simulink model "ControllerSimulation"  (R2024a)
settings: Solver=ode45  StartTime=0.0  StopTime=400  RelTol=1e-4
values from neighbouring files (symbols this model uses):
  CpData = [-0.257802999755 -0.378175309838 -0.529522344065 -0.715215887549 -0.938397956285 -1.2018891109 -1.50731652217 -1.85573677772 -2.24586115735 -2.67483575128 -3.1476672426 -3.67843934333 ... (915 elements, 15x61)]    [WindCpData.mat]
undefined symbols (not defined in the file or in its folder): GBEff, GBRatio, GenEff, J_r, K_theta, PRated, R, rho, T_theta, tau, tau_T, WindRated, wRatedLSS
libraries: simulink x2
settings Model: Creator=The MathWorks, Inc.  LastModifiedBy=alber
settings OptimizationCC: ReuseModelBlockBuffer=off
settings DebuggingCC: SubsystemReferenceDiagnosticForUnitTest=warning
settings RTWCC: GPUComputeCapability=3.5

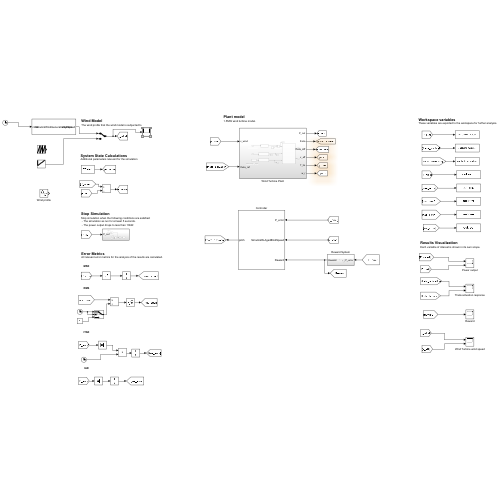
[thumbnail: Simulink's stored preview of the top-level diagram]
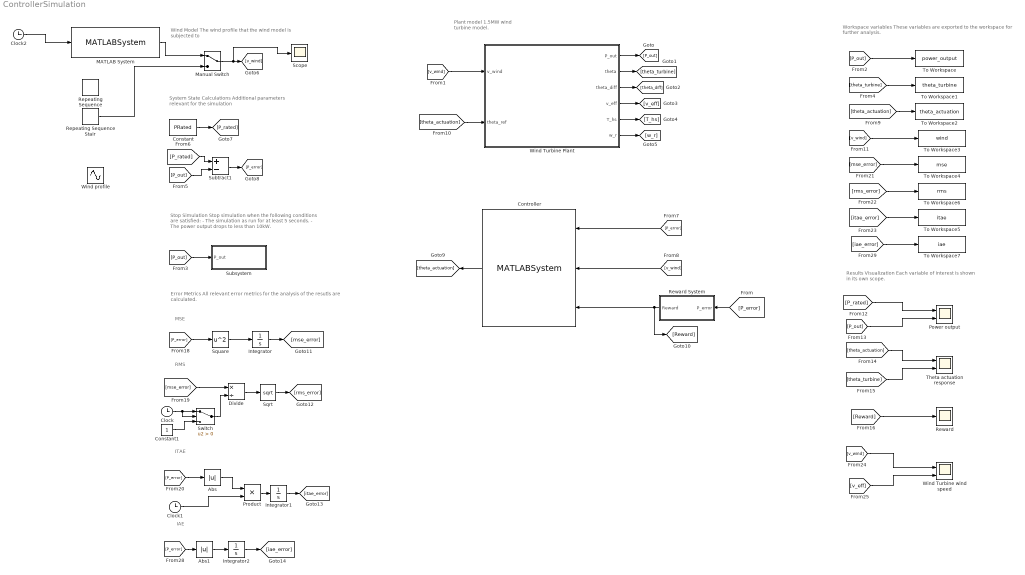
== system ControllerSimulation ==
  note: IAE
  note: MSE
  note: Error Metrics
      | All relevant error metrics for the analysis of the resutls are calculated.
  note: Results Visualization
      | Each variable of interest is shown in its own scope.
  note: System State Calculations
      | Additional parameters relevant for the simulation
  note: Wind Model
      | The wind profile that the wind model is subjected to
  note: Workspace variables
      | These variables are exported to the workspace for further analysis.
  note: Stop Simulation
      | Stop simulation when the following conditions are satisfied:
      | - The simulation as run for at least 5 seconds.
      | - The power output drops to less than 10kW.
  note: Plant model
      | 1.5MW wind turbine model.
  note: RMS
  note: ITAE
  Abs : Abs  SaturateOnIntegerOverflow=off
  Abs1 : Abs  SaturateOnIntegerOverflow=off
  Clock : Clock
  Clock1 : Clock
  Clock2 : Clock
  Constant : Constant  Value=PRated
  Constant1 : Constant
  Controller : MATLABSystem  System=SimulinkRLAgent  SimulateUsing=Interpreted execution
      mask Type: SimulinkRLAgent
      mask Display:
      | disp('SimulinkRLAgent');
      | port_label('input',1,'P_error');
      | port_label('input',2,'WindSpeed');
      | port_label('input',3,'Reward');
      | port_label('output',1,'pitch');
  Divide : Product  Inputs=*/
  Integrator : Integrator
  Integrator1 : Integrator
  Integrator2 : Integrator
  MATLAB System : MATLABSystem  System=SimulinkWindGeneratorSystem  Scale=11.7  Shape=120  Tau=1  MaxRate=0.9  Ts=1  RandomTime=5  SimulateUsing=Interpreted execution
      mask Type: SimulinkWindGeneratorSystem
      mask Display:
      | disp('SimulinkWindGeneratorSystem');
      | port_label('input',1,'clock');
      | port_label('output',1,'windSpeed');
  Manual Switch : ManualSwitch
  Power output : Scope  NumInputPorts=2
  Product : Product
  Repeating Sequence : simulink/Sources/Repeating Sequence  rep_seq_t=[0 401]  rep_seq_y=[11.3 11.9]
  Repeating Sequence Stair : simulink/Sources/Repeating Sequence Stair  OutValues=11.3:0.05:11.9  tsamp=15  OutMin=[11.3]  OutMax=[11.9]  OutDataTypeStr=double  OutputDataTypeScalingMode=double  OutDataType=fixdt(0,8)  ConRadixGroup=Best Precision: Vector-wise  OutScaling=2^-12
  Reward : Scope
  Reward System : Subsystem
  Scope : Scope
  Sqrt : Sqrt
  Square : Math  Operator=square
  Subsystem : Subsystem
  Subtract1 : Sum  Inputs=+-
  Switch : Switch  Criteria=u2 > Threshold  SaturateOnIntegerOverflow=off  InputSameDT=off
  Theta actuation response : Scope  NumInputPorts=2
  To Workspace : ToWorkspace  VariableName=power_output  SaveFormat=Timeseries  SampleTime=-1
  To Workspace1 : ToWorkspace  VariableName=theta_turbine  SaveFormat=Timeseries  SampleTime=-1
  To Workspace2 : ToWorkspace  VariableName=theta_actuation  SaveFormat=Timeseries  SampleTime=-1
  To Workspace3 : ToWorkspace  VariableName=wind  SaveFormat=Timeseries  SampleTime=-1
  To Workspace4 : ToWorkspace  VariableName=mse  SaveFormat=Timeseries  SampleTime=-1
  To Workspace5 : ToWorkspace  VariableName=itae  SaveFormat=Timeseries  SampleTime=-1
  To Workspace6 : ToWorkspace  VariableName=rms  SaveFormat=Timeseries  SampleTime=-1
  To Workspace7 : ToWorkspace  VariableName=iae  SaveFormat=Timeseries  SampleTime=-1
  Wind Turbine Plant : Subsystem
  Wind Turbine wind speed : Scope  NumInputPorts=2
  Wind profile : Sin  Amplitude=.2  Bias=WindRated+0.4  Frequency=0.05  SampleTime=0
  wires:
  Wind Turbine Plant/1(P_out) -> [P_out]
  Wind Turbine Plant/2(theta) -> [theta_turbine]
  Wind Turbine Plant/3(theta_diff) -> [theta_diff]
  Wind Turbine Plant/4(v_eff) -> [v_eff]
  Wind Turbine Plant/5(T_hs) -> [T_hs]
  Wind Turbine Plant/6(w_r) -> [w_r]
  [v_wind] -> Wind Turbine Plant/1(v_wind)
  [P_out] -> To Workspace/1
  [P_out] -> Subsystem/1(P_out)
  [theta_turbine] -> To Workspace1/1
  Constant/1 -> [P_rated]
  [P_rated] -> Subtract1/1
  [P_out] -> Subtract1/2
  Subtract1/1 -> [P_error]
  [P_error] -> Controller/1
  [v_wind] -> Controller/2
  [theta_actuation] -> To Workspace2/1
  Controller/1 -> [theta_actuation]
  [P_error] -> Reward System/1(P_error)
  [v_wind] -> To Workspace3/1
  [P_rated] -> Power output/1
  [P_out] -> Power output/2
  [theta_actuation] -> Theta actuation response/1
  [theta_turbine] -> Theta actuation response/2
  [Reward] -> Reward/1
  [P_error] -> Square/1
  Square/1 -> Integrator/1
  Integrator/1 -> [mse_error]
  [mse_error] -> Divide/1
  Clock/1 -> Switch/2, Switch/1
  Constant1/1 -> Switch/3
  Switch/1 -> Divide/2
  Divide/1 -> Sqrt/1
  Sqrt/1 -> [rms_error]
  [P_error] -> Abs/1
  Abs/1 -> Product/1
  Clock1/1 -> Product/2
  Product/1 -> Integrator1/1
  Integrator1/1 -> [itae_error]
  [mse_error] -> To Workspace4/1
  [rms_error] -> To Workspace6/1
  [itae_error] -> To Workspace5/1
  [v_wind] -> Wind Turbine wind speed/1
  [v_eff] -> Wind Turbine wind speed/2
  [P_error] -> Abs1/1
  Abs1/1 -> Integrator2/1
  Integrator2/1 -> [iae_error]
  [iae_error] -> To Workspace7/1
  [theta_actuation] -> Wind Turbine Plant/2(theta_ref)
  Reward System/1(Reward) -> [Reward], Controller/3
  Manual Switch/1 -> Scope/1, [v_wind]
  MATLAB System/1 -> Manual Switch/1
  Clock2/1 -> MATLAB System/1
  Repeating Sequence Stair/1 -> Manual Switch/2

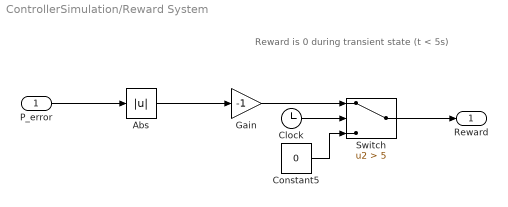
== system ControllerSimulation/Reward System ==
  note: Reward is 0 during transient state (t < 5s)
  P_error : Inport
  Abs : Abs  SaturateOnIntegerOverflow=off
  Clock : Clock
  Constant5 : Constant  Value=0
  Gain : Gain  Gain=-1
  Switch : Switch  Criteria=u2 > Threshold  Threshold=5  SaturateOnIntegerOverflow=off  InputSameDT=off
  Reward : Outport
  wires:
  P_error/1 -> Abs/1
  Clock/1 -> Switch/2
  Gain/1 -> Switch/1
  Constant5/1 -> Switch/3
  Switch/1 -> Reward/1
  Abs/1 -> Gain/1

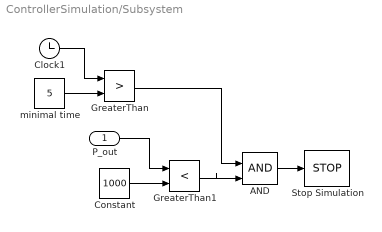
== system ControllerSimulation/Subsystem ==
  P_out : Inport
  AND : Logic  IconShape=distinctive  AllPortsSameDT=off  OutDataTypeStr=boolean
  Clock1 : Clock
  Constant : Constant  Value=1000
  GreaterThan : RelationalOperator  Operator=>  OutDataTypeStr=boolean  RndMeth=Simplest  InputSameDT=off
  GreaterThan1 : RelationalOperator  Operator=<  OutDataTypeStr=boolean  RndMeth=Simplest  InputSameDT=off
  Stop Simulation : Stop
  minimal time : Constant  Value=5
  wires:
  minimal time/1 -> GreaterThan/2
  AND/1 -> Stop Simulation/1
  Constant/1 -> GreaterThan1/2
  GreaterThan1/1 -> AND/2
  GreaterThan/1 -> AND/1
  Clock1/1 -> GreaterThan/1
  P_out/1 -> GreaterThan1/1

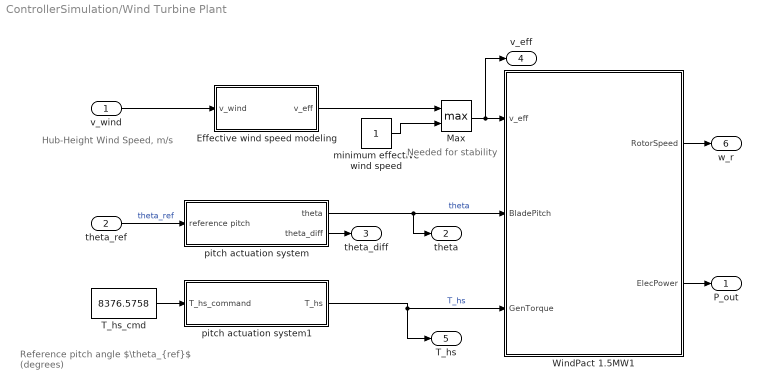
== system ControllerSimulation/Wind Turbine Plant ==
  note: Needed for stability
  note: Hub-Height Wind Speed, m/s
  note: Reference pitch angle $\theta_{ref}$ (degrees)
  v_wind : Inport
  theta_ref : Inport  Port=2
  Effective wind speed modeling : Subsystem
  Max : MinMax  Function=max  Inputs=2
  T_hs_cmd : Constant  Value=8376.5758
  WindPact 1.5MW1 : Subsystem
  minimum effective wind speed : Constant
  pitch actuation system : Subsystem
  pitch actuation system1 : Subsystem
  P_out : Outport
  theta : Outport  Port=2
  theta_diff : Outport  Port=3
  v_eff : Outport  Port=4
  T_hs : Outport  Port=5
  w_r : Outport  Port=6
  wires:
  minimum effective wind speed/1 -> Max/2
  Max/1 -> v_eff/1, WindPact 1.5MW1/1(v_eff)
  Effective wind speed modeling/1(v_eff) -> Max/1
  v_wind/1 -> Effective wind speed modeling/1(v_wind)
  theta_ref/1 -> pitch actuation system/1(reference pitch)  "theta_ref"
  WindPact 1.5MW1/2(ElecPower) -> P_out/1
  pitch actuation system/1(theta) -> WindPact 1.5MW1/2(BladePitch), theta/1  "theta"
  WindPact 1.5MW1/1("RotorSpeed ") -> w_r/1
  pitch actuation system/2(theta_diff) -> theta_diff/1
  T_hs_cmd/1 -> pitch actuation system1/1(T_hs_command)
  pitch actuation system1/1(T_hs) -> WindPact 1.5MW1/3(GenTorque), T_hs/1  "T_hs"

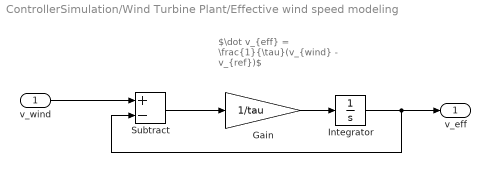
== system ControllerSimulation/Wind Turbine Plant/Effective wind speed modeling ==
  note: $\dot v_{eff} = \frac{1}{\tau}(v_{wind} - v_{ref})$
  v_wind : Inport
  Gain : Gain  Gain=1/tau
  Integrator : Integrator
  Subtract : Sum  Inputs=+-
  v_eff : Outport
  wires:
  Integrator/1 -> Subtract/2, v_eff/1
  Gain/1 -> Integrator/1
  Subtract/1 -> Gain/1
  v_wind/1 -> Subtract/1

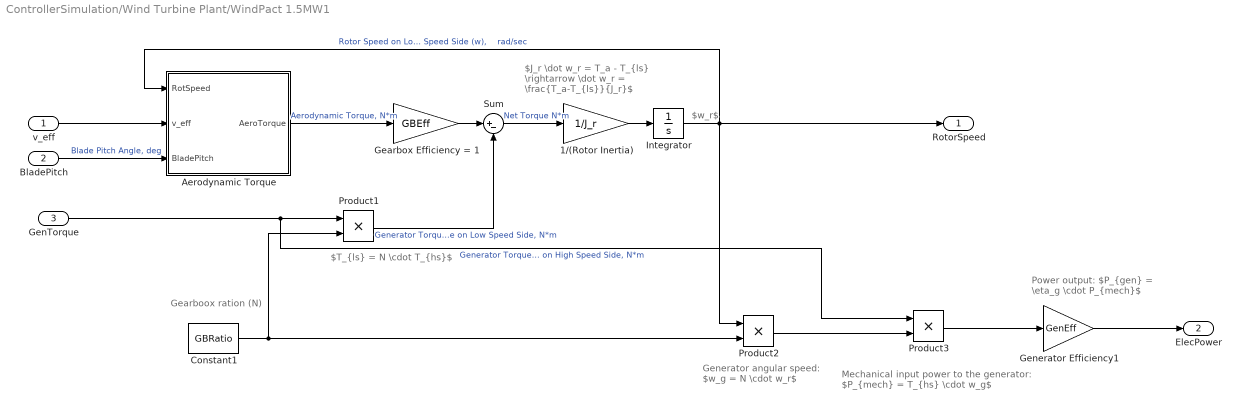
== system ControllerSimulation/Wind Turbine Plant/WindPact 1.5MW1 ==
  note: Gearboox ration (N)
  note: Power output:
      | $P_{gen} = \eta_g \cdot P_{mech}$
  note: Mechanical input power to the generator:
      | $P_{mech} = T_{hs} \cdot w_g$
  note: $w_r$
  note: Generator angular speed:
      | $w_g = N \cdot w_r$
  note: $J_r \dot w_r = T_a - T_{ls} \rightarrow \dot w_r = \frac{T_a-T_{ls}}{J_r}$
  note: $T_{ls} = N \cdot T_{hs}$
  v_eff : Inport
  BladePitch : Inport  Port=2
  GenTorque : Inport  Port=3
  1/(Rotor Inertia) : Gain  Gain=1/J_r
  Aerodynamic Torque : Subsystem
  Constant1 : Constant  Value=GBRatio
  Gearbox Efficiency = 1 : Gain  Gain=GBEff
  Generator Efficiency1 : Gain  Gain=GenEff
  Integrator : Integrator  InitialCondition=wRatedLSS
  Product1 : Product
  Product2 : Product
  Product3 : Product
  Sum : Sum  Inputs=|+-
  "RotorSpeed " : Outport
  ElecPower : Outport  Port=2
  wires:
  Integrator/1 -> "RotorSpeed "/1, Product2/1, Aerodynamic Torque/1("RotSpeed ")  "Rotor Speed on Low Speed Side (w),    rad/sec"
  Sum/1 -> 1/(Rotor Inertia)/1  "Net Torque N*m"
  Gearbox Efficiency = 1/1 -> Sum/1
  Product1/1 -> Sum/2  "Generator Torque on Low Speed Side, N*m"
  1/(Rotor Inertia)/1 -> Integrator/1
  v_eff/1 -> Aerodynamic Torque/2(v_eff)
  GenTorque/1 -> Product3/1, Product1/1  "Generator Torque on High Speed Side, N*m"
  Aerodynamic Torque/1(AeroTorque) -> Gearbox Efficiency = 1/1  "Aerodynamic Torque, N*m"
  BladePitch/1 -> Aerodynamic Torque/3(BladePitch)  "Blade Pitch Angle, deg"
  Constant1/1 -> Product1/2, Product2/2
  Product2/1 -> Product3/2
  Product3/1 -> Generator Efficiency1/1
  Generator Efficiency1/1 -> ElecPower/1

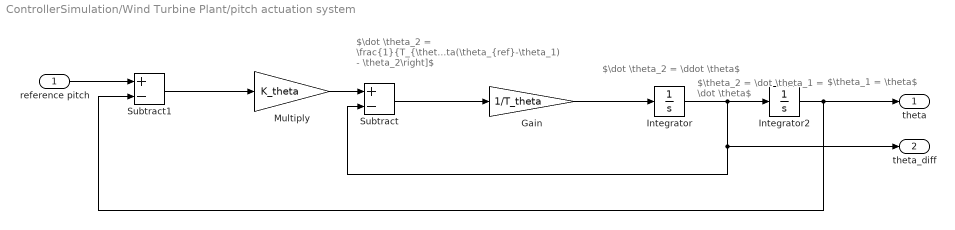
== system ControllerSimulation/Wind Turbine Plant/pitch actuation system ==
  note: $\dot \theta_2 = \frac{1}{T_{\theta}}\left[K_\theta(\theta_{ref}-\theta_1) - \theta_2\right]$
  note: $\theta_1 = \theta$
  note: $\dot \theta_2 = \ddot \theta$
  note: $\theta_2 = \dot \theta_1 = \dot \theta$
  reference pitch : Inport
  Gain : Gain  Gain=1/T_theta
  Integrator : Integrator
  Integrator2 : Integrator
  Multiply : Gain  Gain=K_theta
  Subtract : Sum  Inputs=+-
  Subtract1 : Sum  Inputs=+-
  theta : Outport
  theta_diff : Outport  Port=2
  wires:
  Gain/1 -> Integrator/1
  Multiply/1 -> Subtract/1
  reference pitch/1 -> Subtract1/1
  Subtract1/1 -> Multiply/1
  Subtract/1 -> Gain/1
  Integrator/1 -> theta_diff/1, Subtract/2, Integrator2/1
  Integrator2/1 -> theta/1, Subtract1/2

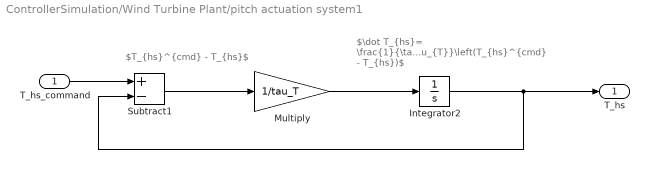
== system ControllerSimulation/Wind Turbine Plant/pitch actuation system1 ==
  note: $T_{hs}^{cmd} - T_{hs}$
  note: $\dot T_{hs}= \frac{1}{\tau_{T}}\left(T_{hs}^{cmd} - T_{hs})$
  T_hs_command : Inport
  Integrator2 : Integrator
  Multiply : Gain  Gain=1/tau_T
  Subtract1 : Sum  Inputs=+-
  T_hs : Outport
  wires:
  Multiply/1 -> Integrator2/1
  T_hs_command/1 -> Subtract1/1
  Subtract1/1 -> Multiply/1
  Integrator2/1 -> Subtract1/2, T_hs/1

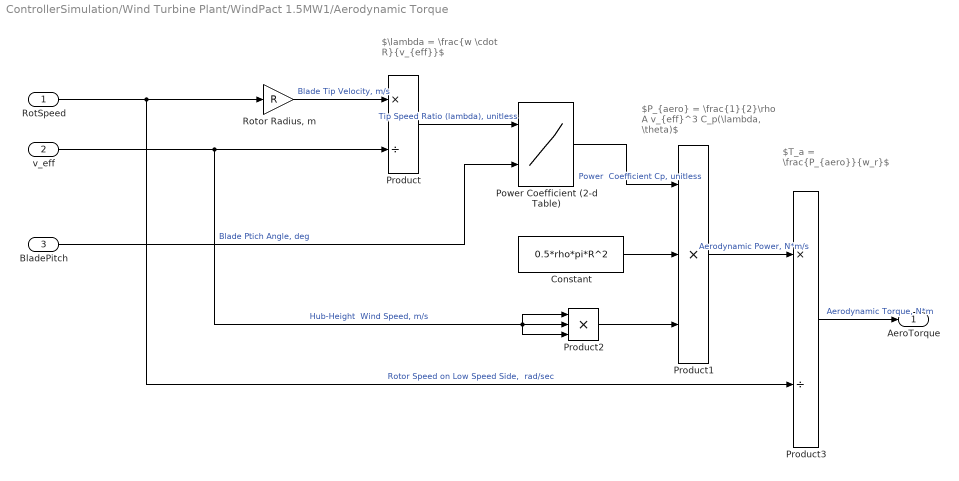
== system ControllerSimulation/Wind Turbine Plant/WindPact 1.5MW1/Aerodynamic Torque ==
  note: $T_a = \frac{P_{aero}}{w_r}$
  note: $\lambda = \frac{w \cdot R}{v_{eff}}$
  note: $P_{aero} = \frac{1}{2}\rho A v_{eff}^3 C_p(\lambda, \theta)$
  "RotSpeed " : Inport
  v_eff : Inport  Port=2
  BladePitch : Inport  Port=3
  Constant : Constant  Value=0.5*rho*pi*R^2
  Power Coefficient (2-d Table) : Lookup2D  RowIndex=TSRgrid  ColumnIndex=Bgrid  Table=CpData  SaturateOnIntegerOverflow=off  InputSameDT=off
  Product : Product  Inputs=*/
  Product1 : Product  Inputs=***
  Product2 : Product  Inputs=***
  Product3 : Product  Inputs=*/
  "Rotor Radius, m" : Gain  Gain=R
  AeroTorque : Outport
  wires:
  "RotSpeed "/1 -> Product3/2, "Rotor Radius, m"/1  "Rotor Speed on Low Speed Side,  rad/sec"
  "Rotor Radius, m"/1 -> Product/1  "Blade Tip Velocity, m/s"
  v_eff/1 -> Product2/3, Product2/1, Product2/2, Product/2  "Hub-Height  Wind Speed, m/s"
  Product/1 -> Power Coefficient (2-d Table)/1  "Tip Speed Ratio (lambda), unitless"
  Power Coefficient (2-d Table)/1 -> Product1/1  "Power  Coefficient Cp, unitless"
  Constant/1 -> Product1/2
  Product2/1 -> Product1/3
  Product1/1 -> Product3/1  "Aerodynamic Power, N*m/s"
  Product3/1 -> AeroTorque/1  "Aerodynamic Torque, N*m"
  BladePitch/1 -> Power Coefficient (2-d Table)/2  "Blade Ptich Angle, deg"
